simulink model "idsm_first_order"  (R2023a)
settings: Solver=FixedStepDiscrete  StartTime=0.0  StopTime=64  FixedStep=1  RelTol=1e-3
undefined symbols (not defined in the file or in its folder): DiscIntNeverNeededParam
settings Model: Creator=bmurm  LastModifiedBy=bmurm

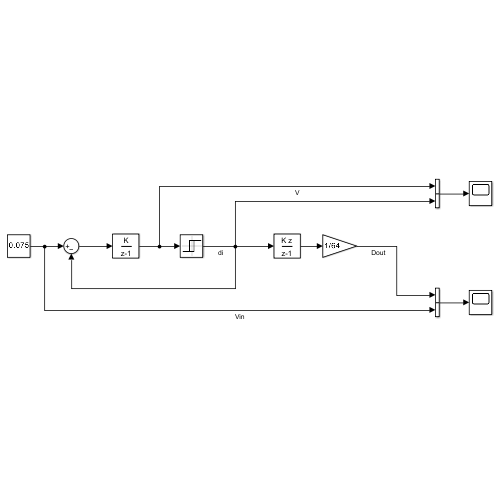
[thumbnail: Simulink's stored preview of the top-level diagram]
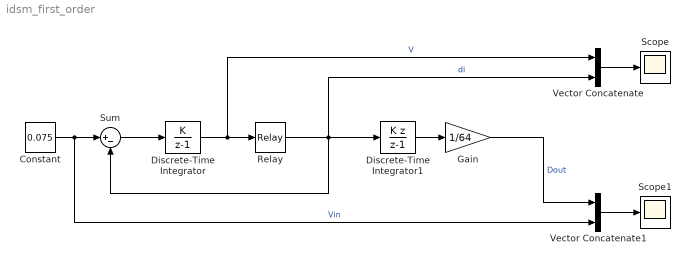
== system idsm_first_order ==
  Constant : Constant  Value=0.075
  Discrete-Time Integrator : DiscreteIntegrator  IntegratorMethod=Accumulation: Forward Euler  SampleTime=-1  ICPrevOutput=DiscIntNeverNeededParam  ICPrevScaledInput=DiscIntNeverNeededParam
  Discrete-Time Integrator1 : DiscreteIntegrator  IntegratorMethod=Accumulation: Backward Euler  SampleTime=-1  ICPrevOutput=DiscIntNeverNeededParam  ICPrevScaledInput=DiscIntNeverNeededParam
  Gain : Gain  Gain=1/64
  Relay : Relay
  Scope : Scope
  Scope1 : Scope
  Sum : Sum  Inputs=|+-
  Vector Concatenate : Concatenate
  Vector Concatenate1 : Concatenate
  wires:
  Sum/1 -> Discrete-Time Integrator/1
  Discrete-Time Integrator/1 -> Vector Concatenate/1, Relay/1  "V"
  Relay/1 -> Discrete-Time Integrator1/1, Vector Concatenate/2, Sum/2  "di"
  Vector Concatenate/1 -> Scope/1
  Constant/1 -> Vector Concatenate1/2, Sum/1  "Vin"
  Vector Concatenate1/1 -> Scope1/1
  Discrete-Time Integrator1/1 -> Gain/1
  Gain/1 -> Vector Concatenate1/1  "Dout"
